simulink model "ScriptDemo"  (R2022b)
settings: configuration reference "TmVcThermal_Configuration_sub" (kept outside this file)
undefined symbols (not defined in the file): aaaa, bbbb, cTmComprCtrl_D_u8HvacFlowTable_db, cTmComprCtrl_D_u8HvacFlowTable_sw, cTmComprCtrl_n_i16ChillCmpIMax, cTmComprCtrl_n_i16ChillCmpIMin, cTmComprCtrl_n_i16ChillCmpIMin666, cTmComprCtrl_n_i16ChillCmpPMax, cTmComprCtrl_n_i16ChillCmpPMin, cTmComprCtrl_n_i16CmpChillCoolRpmKiMax, cTmComprCtrl_n_i16CmpChillCoolRpmKiMin, cTmComprCtrl_n_i16CmpChillCoolRpmKpMax, cTmComprCtrl_n_i16CmpChillCoolRpmKpMin, cTmComprCtrl_n_i16CmpCoolRpmKiMax, cTmComprCtrl_n_i16CmpCoolRpmKiMin, cTmComprCtrl_n_i16CmpCoolRpmKpMax, cTmComprCtrl_n_i16CmpCoolRpmKpMin, cTmComprCtrl_n_i16SM4CmpHeatKiMax, cTmComprCtrl_n_i16SM4CmpHeatKiMin, cTmComprCtrl_n_i16SM4CmpHeatKpMax, cTmComprCtrl_n_i16SM4CmpHeatKpMin, cTmComprCtrl_n_i16SM5CmpHeatKiMax, cTmComprCtrl_n_i16SM5CmpHeatKiMin, cTmComprCtrl_n_i16SM5CmpHeatKpMax, cTmComprCtrl_n_i16SM5CmpHeatKpMin, cTmComprCtrl_n_i16SM6CmpHeatKiMax, cTmComprCtrl_n_i16SM6CmpHeatKiMin, cTmComprCtrl_n_i16SM6CmpHeatKpMax, cTmComprCtrl_n_i16SM6CmpHeatKpMin, cTmComprCtrl_n_u16CmpMaxSpdFanFltLimt, cTmComprCtrl_n_u16CmpMaxSpdLoSidePFltLimt, cTmComprCtrl_n_u16CmpMaxSpdSensorFltLimt, cTmComprCtrl_n_u16CompMinRpm, cTmComprCtrl_n_u16CompRpmIncThres, cTmComprCtrl_t_u16BattCooltFFPeriod, cTmComprCtrl_t_u16BattCooltPIPeriod, cTmComprCtrl_t_u16CmpCoolFFPeriod, cTmComprCtrl_t_u16CmpCoolPIPeriod, cTmComprCtrl_t_u16CoolCmpChillFFPeriod, cTmComprCtrl_t_u16CoolCmpChillPIPeriod, cTmComprCtrl_t_u16SM4CmpHeatFFPeriod, cTmComprCtrl_t_u16SM4CmpHeatPIPeriod, cTmComprCtrl_t_u16SM5CmpHeatFFPeriod, cTmComprCtrl_t_u16SM5CmpHeatPIPeriod, cTmComprCtrl_t_u16SM6CmpHeatFFPeriod, cTmComprCtrl_t_u16SM6CmpHeatPIPeriod, cTmComprCtrl_Te_EvapClearInteg, cTmComprCtrl_Te_i16HpReqTempSaturoffset, cTmComprCtrl_Te_i16SatLpReplaceDiff, cTmComprCtrl_Te_i16SM3BatDiffStartEvapDecOffset, cTmComprCtrl_Te_i16SM3EvapLo, cTmComprCtrl_Te_i16SM3TBatDiffEntEvapDecOffset, cTmComprCtrl_Te_i16SM3TBatDiffEntEvapDecOffsetQuit, cTmComprCtrl_Te_s32ErrCmpChillPIContinueCoolH, cTmComprCtrl_Te_s32ErrCmpChillPIContinueCoolL, cTmComprCtrl_Te_s32ErrCmpPIContinueChillH, cTmComprCtrl_Te_s32ErrCmpPIContinueChillL, cTmComprCtrl_Te_s32ErrCmpPIContinueCoolH, cTmComprCtrl_Te_s32ErrCmpPIContinueCoolL, cTmComprCtrl_Te_s32ErrCmpPIContinueHeatH ... (+398)
libraries: simulink x782, PCMULib x640, simulink_need_slupdate x4
(part 9 of 41)

== system ScriptDemo/Create/Model/createModGotoAll/After ==
  note: createModGotoAll()
      |
      | # 在此路径下执行
  AFFaultLimit : Subsystem
  LoSidePFltLimt : Subsystem
  SensFaultLimit : Subsystem
  TAmbLimit : Subsystem
  wires:
  [sTmDiag_D_u8FanFltSt] -> AFFaultLimit/1(sTmDiag_D_u8FanFltSt)
  AFFaultLimit/1(rTmComprCtrl_n_u16CompMaxRpmAfFlt) -> [rTmComprCtrl_n_u16CompMaxRpmAfFlt]
  AFFaultLimit/2(xTmComprCtrl_B_CmpFanFltLimtFlag) -> [xTmComprCtrl_B_CmpFanFltLimtFlag]
  [sTmDiag_D_u8LoSidePFltSt] -> LoSidePFltLimt/1(sTmDiag_D_u8LoSidePFltSt)
  [sTmSigProces_Te_s32TAmb] -> LoSidePFltLimt/2(sTmSigProces_Te_s32TAmb)
  [sTmIn_D_u8HeatPump] -> LoSidePFltLimt/3(sTmIn_D_u8HeatPump)
  LoSidePFltLimt/1(rTmComprCtrl_n_u16CompMaxRpmLoSidePFlt) -> [rTmComprCtrl_n_u16CompMaxRpmLoSidePFlt]
  LoSidePFltLimt/2(xTmComprCtrl_B_CmpLoSidePFltLimtFlag) -> [xTmComprCtrl_B_CmpLoSidePFltLimtFlag]
  [sTmDiag_D_u8CmprDischrgTFltSt] -> SensFaultLimit/1(sTmDiag_D_u8CmprDischrgTFltSt)
  [sTmDiag_D_u8HiSidePFltSt] -> SensFaultLimit/2(sTmDiag_D_u8HiSidePFltSt)
  [sTmDiag_D_u8OutrCondOutTFltSt] -> SensFaultLimit/3(sTmDiag_D_u8OutrCondOutTFltSt)
  [sTmIn_D_u8HeatPump] -> SensFaultLimit/4(sTmIn_D_u8HeatPump)
  [sTmDiag_D_u8HiSidePNHPFltSt] -> SensFaultLimit/5(sTmDiag_D_u8HiSidePNHPFltSt)
  SensFaultLimit/1(rTmComprCtrl_n_u16CompMaxRpmSensFlt) -> [rTmComprCtrl_n_u16CompMaxRpmSensFlt]
  SensFaultLimit/2(xTmComprCtrl_B_CmpSensorFltLimtFlag) -> [xTmComprCtrl_B_CmpSensorFltLimtFlag]
  [sTmSigProces_Pw_i16ReqPwrForHeat] -> TAmbLimit/1(sTmSigProces_Pw_i16ReqPwrForHeat)
  [sTmSigProces_Te_s32TAmb] -> TAmbLimit/2(sTmSigProces_Te_s32TAmb)
  [rTmComprCtrl_n_u16CompRpmReqBoundary] -> TAmbLimit/3(rTmComprCtrl_n_u16CompRpmReqBoundary)
  [sTmRefriModeMgr_D_u8HPCurMode] -> TAmbLimit/4(sTmRefriModeMgr_D_u8HPCurMode)
  TAmbLimit/1(rTmComprCtrl_n_u16CompMaxRpmTAmb) -> [rTmComprCtrl_n_u16CompMaxRpmTAmb]
  TAmbLimit/2(xTmComprCtrl_B_CmpAmbLimtFlag) -> [xTmComprCtrl_B_CmpAmbLimtFlag]

== system ScriptDemo/Create/Model/createModGotoAll/Before ==
  AFFaultLimit : Subsystem
  LoSidePFltLimt : Subsystem
  SensFaultLimit : Subsystem
  TAmbLimit : Subsystem

== system ScriptDemo/Create/Model/createModGroundTerm/After ==
  note: % 目的: 为输出端口创建debug 及对应的输入模块
      | [cnt] = createDebug(gcs)
  sTmRefriVlvCtrl_X_s32CEXVPosReqIn : Inport  OutDataTypeStr=single
  sTmRefriVlvCtrl_X_s32EEXVPosReqIn : Inport  Port=2  OutDataTypeStr=single
  sTmRefriVlvCtrl_X_s32BEXVPosReqIn : Inport  Port=3  OutDataTypeStr=single
  yTmRefriVlvCtrl_B_HpcCexvMovEnableIn : Inport  Port=4  OutDataTypeStr=boolean
  sTmRefriVlvCtrl_Z_u8CEXVInitStateIn : Inport  Port=5  OutDataTypeStr=uint8
  yTmRefriVlvCtrl_B_CexvCalibReqIn : Inport  Port=6  OutDataTypeStr=boolean
  yTmRefriVlvCtrl_B_HpcEexvMovEnableIn : Inport  Port=7  OutDataTypeStr=boolean
  sTmRefriVlvCtrl_Z_u8EEXVInitStateIn : Inport  Port=8  OutDataTypeStr=uint8
  yTmRefriVlvCtrl_B_EexvCalibReqIn : Inport  Port=9  OutDataTypeStr=boolean
  yTmRefriVlvCtrl_B_HpcBexvMovEnableIn : Inport  Port=10  OutDataTypeStr=boolean
  sTmRefriVlvCtrl_Z_u8BEXVInitStateIn : Inport  Port=11  OutDataTypeStr=uint8
  yTmRefriVlvCtrl_B_BexvCalibReqIn : Inport  Port=12  OutDataTypeStr=boolean
  sTmRefriVlvCtrl_X_s32SM3BexvMaxPosIn : Inport  Port=13  OutDataTypeStr=single
  yTmRefriVlvCtrl_B_EvapBattTLimBexvEnaIn : Inport  Port=14  OutDataTypeStr=boolean
  sTmRefriVlvCtrl_D_u8EexvRefriSwitchStIn : Inport  Port=15  OutDataTypeStr=uint8
  sTmRefriVlvCtrl_D_u8CexvRefriSwitchStIn : Inport  Port=16  OutDataTypeStr=uint8
  sTmRefriVlvCtrl_D_u8BexvRefriSwitchStIn : Inport  Port=17  OutDataTypeStr=uint8
  OutDebug : PCMULib/Interface/OutdebugRvs  SWI=cTmRefriVlvCtrl_X_s32CEXVPosReq_sw  DBI=cTmRefriVlvCtrl_X_s32CEXVPosReq_db
      settings: SourceProductName=PCMULib
  OutDebug1 : PCMULib/Interface/OutdebugRvs  SWI=cTmRefriVlvCtrl_X_s32EEXVPosReq_sw  DBI=cTmRefriVlvCtrl_X_s32EEXVPosReq_db
      settings: SourceProductName=PCMULib
  OutDebug10 : PCMULib/Interface/OutdebugRvs  SWI=cTmRefriVlvCtrl_Z_u8BEXVInitState_sw  DBI=cTmRefriVlvCtrl_Z_u8BEXVInitState_db
      settings: SourceProductName=PCMULib
  OutDebug11 : PCMULib/Interface/OutdebugRvs  SWI=cTmRefriVlvCtrl_B_BexvCalibReq_sw  DBI=cTmRefriVlvCtrl_B_BexvCalibReq_db
      settings: SourceProductName=PCMULib
  OutDebug12 : PCMULib/Interface/OutdebugRvs  SWI=cTmRefriVlvCtrl_X_s32SM3BexvMaxPos_sw  DBI=cTmRefriVlvCtrl_X_s32SM3BexvMaxPos_db
      settings: SourceProductName=PCMULib
  OutDebug13 : PCMULib/Interface/OutdebugRvs  SWI=cTmRefriVlvCtrl_B_EvapBattTLimBexvEna_sw  DBI=cTmRefriVlvCtrl_B_EvapBattTLimBexvEna_db
      settings: SourceProductName=PCMULib
  OutDebug14 : PCMULib/Interface/OutdebugRvs  SWI=cTmRefriVlvCtrl_D_u8EexvRefriSwitchSt_sw  DBI=cTmRefriVlvCtrl_D_u8EexvRefriSwitchSt_db
      settings: SourceProductName=PCMULib
  OutDebug15 : PCMULib/Interface/OutdebugRvs  SWI=cTmRefriVlvCtrl_D_u8CexvRefriSwitchSt_sw  DBI=cTmRefriVlvCtrl_D_u8CexvRefriSwitchSt_db
      settings: SourceProductName=PCMULib
  OutDebug16 : PCMULib/Interface/OutdebugRvs  SWI=cTmRefriVlvCtrl_D_u8BexvRefriSwitchSt_sw  DBI=cTmRefriVlvCtrl_D_u8BexvRefriSwitchSt_db
      settings: SourceProductName=PCMULib
  OutDebug2 : PCMULib/Interface/OutdebugRvs  SWI=cTmRefriVlvCtrl_X_s32BEXVPosReq_sw  DBI=cTmRefriVlvCtrl_X_s32BEXVPosReq_db
      settings: SourceProductName=PCMULib
  OutDebug3 : PCMULib/Interface/OutdebugRvs  SWI=cTmRefriVlvCtrl_B_HpcCexvMovEnable_sw  DBI=cTmRefriVlvCtrl_B_HpcCexvMovEnable_db
      settings: SourceProductName=PCMULib
  OutDebug4 : PCMULib/Interface/OutdebugRvs  SWI=cTmRefriVlvCtrl_Z_u8CEXVInitState_sw  DBI=cTmRefriVlvCtrl_Z_u8CEXVInitState_db
      settings: SourceProductName=PCMULib
  OutDebug5 : PCMULib/Interface/OutdebugRvs  SWI=cTmRefriVlvCtrl_B_CexvCalibReq_sw  DBI=cTmRefriVlvCtrl_B_CexvCalibReq_db
      settings: SourceProductName=PCMULib
  OutDebug6 : PCMULib/Interface/OutdebugRvs  SWI=cTmRefriVlvCtrl_B_HpcEexvMovEnable_sw  DBI=cTmRefriVlvCtrl_B_HpcEexvMovEnable_db
      settings: SourceProductName=PCMULib
  OutDebug7 : PCMULib/Interface/OutdebugRvs  SWI=cTmRefriVlvCtrl_Z_u8EEXVInitState_sw  DBI=cTmRefriVlvCtrl_Z_u8EEXVInitState_db
      settings: SourceProductName=PCMULib
  OutDebug8 : PCMULib/Interface/OutdebugRvs  SWI=cTmRefriVlvCtrl_B_EexvCalibReq_sw  DBI=cTmRefriVlvCtrl_B_EexvCalibReq_db
      settings: SourceProductName=PCMULib
  OutDebug9 : PCMULib/Interface/OutdebugRvs  SWI=cTmRefriVlvCtrl_B_HpcBexvMovEnable_sw  DBI=cTmRefriVlvCtrl_B_HpcBexvMovEnable_db
      settings: SourceProductName=PCMULib
  sTmRefriVlvCtrl_X_s32CEXVPosReq : Outport  OutDataTypeStr=single
  sTmRefriVlvCtrl_X_s32EEXVPosReq : Outport  Port=2  OutDataTypeStr=single
  sTmRefriVlvCtrl_X_s32BEXVPosReq : Outport  Port=3  OutDataTypeStr=single
  yTmRefriVlvCtrl_B_HpcCexvMovEnable : Outport  Port=4  OutDataTypeStr=boolean
  sTmRefriVlvCtrl_Z_u8CEXVInitState : Outport  Port=5  OutDataTypeStr=uint8
  yTmRefriVlvCtrl_B_CexvCalibReq : Outport  Port=6  OutDataTypeStr=boolean
  yTmRefriVlvCtrl_B_HpcEexvMovEnable : Outport  Port=7  OutDataTypeStr=boolean
  sTmRefriVlvCtrl_Z_u8EEXVInitState : Outport  Port=8  OutDataTypeStr=uint8
  yTmRefriVlvCtrl_B_EexvCalibReq : Outport  Port=9  OutDataTypeStr=boolean
  yTmRefriVlvCtrl_B_HpcBexvMovEnable : Outport  Port=10  OutDataTypeStr=boolean
  sTmRefriVlvCtrl_Z_u8BEXVInitState : Outport  Port=11  OutDataTypeStr=uint8
  yTmRefriVlvCtrl_B_BexvCalibReq : Outport  Port=12  OutDataTypeStr=boolean
  sTmRefriVlvCtrl_X_s32SM3BexvMaxPos : Outport  Port=13  OutDataTypeStr=single
  yTmRefriVlvCtrl_B_EvapBattTLimBexvEna : Outport  Port=14  OutDataTypeStr=boolean
  sTmRefriVlvCtrl_D_u8EexvRefriSwitchSt : Outport  Port=15  OutDataTypeStr=uint8
  sTmRefriVlvCtrl_D_u8CexvRefriSwitchSt : Outport  Port=16  OutDataTypeStr=uint8
  sTmRefriVlvCtrl_D_u8BexvRefriSwitchSt : Outport  Port=17  OutDataTypeStr=uint8
  wires:
  sTmRefriVlvCtrl_X_s32SM3BexvMaxPosIn/1 -> OutDebug12/1
  OutDebug12/1 -> sTmRefriVlvCtrl_X_s32SM3BexvMaxPos/1
  sTmRefriVlvCtrl_X_s32BEXVPosReqIn/1 -> OutDebug2/1
  OutDebug2/1 -> sTmRefriVlvCtrl_X_s32BEXVPosReq/1
  OutDebug16/1 -> sTmRefriVlvCtrl_D_u8BexvRefriSwitchSt/1
  sTmRefriVlvCtrl_D_u8EexvRefriSwitchStIn/1 -> OutDebug14/1
  OutDebug5/1 -> yTmRefriVlvCtrl_B_CexvCalibReq/1
  OutDebug3/1 -> yTmRefriVlvCtrl_B_HpcCexvMovEnable/1
  sTmRefriVlvCtrl_Z_u8CEXVInitStateIn/1 -> OutDebug4/1
  OutDebug4/1 -> sTmRefriVlvCtrl_Z_u8CEXVInitState/1
  sTmRefriVlvCtrl_D_u8BexvRefriSwitchStIn/1 -> OutDebug16/1
  OutDebug1/1 -> sTmRefriVlvCtrl_X_s32EEXVPosReq/1
  OutDebug14/1 -> sTmRefriVlvCtrl_D_u8EexvRefriSwitchSt/1
  yTmRefriVlvCtrl_B_CexvCalibReqIn/1 -> OutDebug5/1
  sTmRefriVlvCtrl_X_s32EEXVPosReqIn/1 -> OutDebug1/1
  yTmRefriVlvCtrl_B_HpcCexvMovEnableIn/1 -> OutDebug3/1
  yTmRefriVlvCtrl_B_EvapBattTLimBexvEnaIn/1 -> OutDebug13/1
  OutDebug13/1 -> yTmRefriVlvCtrl_B_EvapBattTLimBexvEna/1
  sTmRefriVlvCtrl_Z_u8BEXVInitStateIn/1 -> OutDebug10/1
  OutDebug10/1 -> sTmRefriVlvCtrl_Z_u8BEXVInitState/1
  sTmRefriVlvCtrl_D_u8CexvRefriSwitchStIn/1 -> OutDebug15/1
  OutDebug15/1 -> sTmRefriVlvCtrl_D_u8CexvRefriSwitchSt/1
  OutDebug/1 -> sTmRefriVlvCtrl_X_s32CEXVPosReq/1
  OutDebug7/1 -> sTmRefriVlvCtrl_Z_u8EEXVInitState/1
  OutDebug8/1 -> yTmRefriVlvCtrl_B_EexvCalibReq/1
  yTmRefriVlvCtrl_B_EexvCalibReqIn/1 -> OutDebug8/1
  sTmRefriVlvCtrl_X_s32CEXVPosReqIn/1 -> OutDebug/1
  OutDebug6/1 -> yTmRefriVlvCtrl_B_HpcEexvMovEnable/1
  yTmRefriVlvCtrl_B_HpcEexvMovEnableIn/1 -> OutDebug6/1
  sTmRefriVlvCtrl_Z_u8EEXVInitStateIn/1 -> OutDebug7/1
  yTmRefriVlvCtrl_B_HpcBexvMovEnableIn/1 -> OutDebug9/1
  OutDebug9/1 -> yTmRefriVlvCtrl_B_HpcBexvMovEnable/1
  yTmRefriVlvCtrl_B_BexvCalibReqIn/1 -> OutDebug11/1
  OutDebug11/1 -> yTmRefriVlvCtrl_B_BexvCalibReq/1

== system ScriptDemo/Create/Model/createModGroundTerm/Before ==
  note: % 目的: 为输出端口创建debug 及对应的输入模块
      | [cnt] = createDebug(gcs)
  sTmRefriVlvCtrl_X_s32CEXVPosReqIn : Inport  OutDataTypeStr=single
  sTmRefriVlvCtrl_X_s32EEXVPosReqIn : Inport  Port=2  OutDataTypeStr=single
  sTmRefriVlvCtrl_X_s32BEXVPosReqIn : Inport  Port=3  OutDataTypeStr=single
  yTmRefriVlvCtrl_B_HpcCexvMovEnableIn : Inport  Port=4  OutDataTypeStr=boolean
  sTmRefriVlvCtrl_Z_u8CEXVInitStateIn : Inport  Port=5  OutDataTypeStr=uint8
  yTmRefriVlvCtrl_B_CexvCalibReqIn : Inport  Port=6  OutDataTypeStr=boolean
  yTmRefriVlvCtrl_B_HpcEexvMovEnableIn : Inport  Port=7  OutDataTypeStr=boolean
  sTmRefriVlvCtrl_Z_u8EEXVInitStateIn : Inport  Port=8  OutDataTypeStr=uint8
  yTmRefriVlvCtrl_B_EexvCalibReqIn : Inport  Port=9  OutDataTypeStr=boolean
  yTmRefriVlvCtrl_B_HpcBexvMovEnableIn : Inport  Port=10  OutDataTypeStr=boolean
  sTmRefriVlvCtrl_Z_u8BEXVInitStateIn : Inport  Port=11  OutDataTypeStr=uint8
  yTmRefriVlvCtrl_B_BexvCalibReqIn : Inport  Port=12  OutDataTypeStr=boolean
  sTmRefriVlvCtrl_X_s32SM3BexvMaxPosIn : Inport  Port=13  OutDataTypeStr=single
  yTmRefriVlvCtrl_B_EvapBattTLimBexvEnaIn : Inport  Port=14  OutDataTypeStr=boolean
  sTmRefriVlvCtrl_D_u8EexvRefriSwitchStIn : Inport  Port=15  OutDataTypeStr=uint8
  sTmRefriVlvCtrl_D_u8CexvRefriSwitchStIn : Inport  Port=16  OutDataTypeStr=uint8
  sTmRefriVlvCtrl_D_u8BexvRefriSwitchStIn : Inport  Port=17  OutDataTypeStr=uint8
  OutDebug : PCMULib/Interface/OutdebugRvs  SWI=cTmRefriVlvCtrl_X_s32CEXVPosReq_sw  DBI=cTmRefriVlvCtrl_X_s32CEXVPosReq_db
      settings: SourceProductName=PCMULib
  OutDebug1 : PCMULib/Interface/OutdebugRvs  SWI=cTmRefriVlvCtrl_X_s32EEXVPosReq_sw  DBI=cTmRefriVlvCtrl_X_s32EEXVPosReq_db
      settings: SourceProductName=PCMULib
  OutDebug10 : PCMULib/Interface/OutdebugRvs  SWI=cTmRefriVlvCtrl_Z_u8BEXVInitState_sw  DBI=cTmRefriVlvCtrl_Z_u8BEXVInitState_db
      settings: SourceProductName=PCMULib
  OutDebug11 : PCMULib/Interface/OutdebugRvs  SWI=cTmRefriVlvCtrl_B_BexvCalibReq_sw  DBI=cTmRefriVlvCtrl_B_BexvCalibReq_db
      settings: SourceProductName=PCMULib
  OutDebug12 : PCMULib/Interface/OutdebugRvs  SWI=cTmRefriVlvCtrl_X_s32SM3BexvMaxPos_sw  DBI=cTmRefriVlvCtrl_X_s32SM3BexvMaxPos_db
      settings: SourceProductName=PCMULib
  OutDebug13 : PCMULib/Interface/OutdebugRvs  SWI=cTmRefriVlvCtrl_B_EvapBattTLimBexvEna_sw  DBI=cTmRefriVlvCtrl_B_EvapBattTLimBexvEna_db
      settings: SourceProductName=PCMULib
  OutDebug14 : PCMULib/Interface/OutdebugRvs  SWI=cTmRefriVlvCtrl_D_u8EexvRefriSwitchSt_sw  DBI=cTmRefriVlvCtrl_D_u8EexvRefriSwitchSt_db
      settings: SourceProductName=PCMULib
  OutDebug15 : PCMULib/Interface/OutdebugRvs  SWI=cTmRefriVlvCtrl_D_u8CexvRefriSwitchSt_sw  DBI=cTmRefriVlvCtrl_D_u8CexvRefriSwitchSt_db
      settings: SourceProductName=PCMULib
  OutDebug16 : PCMULib/Interface/OutdebugRvs  SWI=cTmRefriVlvCtrl_D_u8BexvRefriSwitchSt_sw  DBI=cTmRefriVlvCtrl_D_u8BexvRefriSwitchSt_db
      settings: SourceProductName=PCMULib
  OutDebug2 : PCMULib/Interface/OutdebugRvs  SWI=cTmRefriVlvCtrl_X_s32BEXVPosReq_sw  DBI=cTmRefriVlvCtrl_X_s32BEXVPosReq_db
      settings: SourceProductName=PCMULib
  OutDebug3 : PCMULib/Interface/OutdebugRvs  SWI=cTmRefriVlvCtrl_B_HpcCexvMovEnable_sw  DBI=cTmRefriVlvCtrl_B_HpcCexvMovEnable_db
      settings: SourceProductName=PCMULib
  OutDebug4 : PCMULib/Interface/OutdebugRvs  SWI=cTmRefriVlvCtrl_Z_u8CEXVInitState_sw  DBI=cTmRefriVlvCtrl_Z_u8CEXVInitState_db
      settings: SourceProductName=PCMULib
  OutDebug5 : PCMULib/Interface/OutdebugRvs  SWI=cTmRefriVlvCtrl_B_CexvCalibReq_sw  DBI=cTmRefriVlvCtrl_B_CexvCalibReq_db
      settings: SourceProductName=PCMULib
  OutDebug6 : PCMULib/Interface/OutdebugRvs  SWI=cTmRefriVlvCtrl_B_HpcEexvMovEnable_sw  DBI=cTmRefriVlvCtrl_B_HpcEexvMovEnable_db
      settings: SourceProductName=PCMULib
  OutDebug7 : PCMULib/Interface/OutdebugRvs  SWI=cTmRefriVlvCtrl_Z_u8EEXVInitState_sw  DBI=cTmRefriVlvCtrl_Z_u8EEXVInitState_db
      settings: SourceProductName=PCMULib
  OutDebug8 : PCMULib/Interface/OutdebugRvs  SWI=cTmRefriVlvCtrl_B_EexvCalibReq_sw  DBI=cTmRefriVlvCtrl_B_EexvCalibReq_db
      settings: SourceProductName=PCMULib
  OutDebug9 : PCMULib/Interface/OutdebugRvs  SWI=cTmRefriVlvCtrl_B_HpcBexvMovEnable_sw  DBI=cTmRefriVlvCtrl_B_HpcBexvMovEnable_db
      settings: SourceProductName=PCMULib
  sTmRefriVlvCtrl_X_s32CEXVPosReq : Outport  OutDataTypeStr=single
  sTmRefriVlvCtrl_X_s32EEXVPosReq : Outport  Port=2  OutDataTypeStr=single
  sTmRefriVlvCtrl_X_s32BEXVPosReq : Outport  Port=3  OutDataTypeStr=single
  yTmRefriVlvCtrl_B_HpcCexvMovEnable : Outport  Port=4  OutDataTypeStr=boolean
  sTmRefriVlvCtrl_Z_u8CEXVInitState : Outport  Port=5  OutDataTypeStr=uint8
  yTmRefriVlvCtrl_B_CexvCalibReq : Outport  Port=6  OutDataTypeStr=boolean
  yTmRefriVlvCtrl_B_HpcEexvMovEnable : Outport  Port=7  OutDataTypeStr=boolean
  sTmRefriVlvCtrl_Z_u8EEXVInitState : Outport  Port=8  OutDataTypeStr=uint8
  yTmRefriVlvCtrl_B_EexvCalibReq : Outport  Port=9  OutDataTypeStr=boolean
  yTmRefriVlvCtrl_B_HpcBexvMovEnable : Outport  Port=10  OutDataTypeStr=boolean
  sTmRefriVlvCtrl_Z_u8BEXVInitState : Outport  Port=11  OutDataTypeStr=uint8
  yTmRefriVlvCtrl_B_BexvCalibReq : Outport  Port=12  OutDataTypeStr=boolean
  sTmRefriVlvCtrl_X_s32SM3BexvMaxPos : Outport  Port=13  OutDataTypeStr=single
  yTmRefriVlvCtrl_B_EvapBattTLimBexvEna : Outport  Port=14  OutDataTypeStr=boolean
  sTmRefriVlvCtrl_D_u8EexvRefriSwitchSt : Outport  Port=15  OutDataTypeStr=uint8
  sTmRefriVlvCtrl_D_u8CexvRefriSwitchSt : Outport  Port=16  OutDataTypeStr=uint8
  sTmRefriVlvCtrl_D_u8BexvRefriSwitchSt : Outport  Port=17  OutDataTypeStr=uint8
  wires:
  sTmRefriVlvCtrl_X_s32SM3BexvMaxPosIn/1 -> OutDebug12/1
  OutDebug12/1 -> sTmRefriVlvCtrl_X_s32SM3BexvMaxPos/1
  sTmRefriVlvCtrl_X_s32BEXVPosReqIn/1 -> OutDebug2/1
  OutDebug2/1 -> sTmRefriVlvCtrl_X_s32BEXVPosReq/1
  OutDebug16/1 -> sTmRefriVlvCtrl_D_u8BexvRefriSwitchSt/1
  sTmRefriVlvCtrl_D_u8EexvRefriSwitchStIn/1 -> OutDebug14/1
  OutDebug5/1 -> yTmRefriVlvCtrl_B_CexvCalibReq/1
  OutDebug3/1 -> yTmRefriVlvCtrl_B_HpcCexvMovEnable/1
  sTmRefriVlvCtrl_Z_u8CEXVInitStateIn/1 -> OutDebug4/1
  OutDebug4/1 -> sTmRefriVlvCtrl_Z_u8CEXVInitState/1
  sTmRefriVlvCtrl_D_u8BexvRefriSwitchStIn/1 -> OutDebug16/1
  OutDebug1/1 -> sTmRefriVlvCtrl_X_s32EEXVPosReq/1
  OutDebug14/1 -> sTmRefriVlvCtrl_D_u8EexvRefriSwitchSt/1
  yTmRefriVlvCtrl_B_CexvCalibReqIn/1 -> OutDebug5/1
  sTmRefriVlvCtrl_X_s32EEXVPosReqIn/1 -> OutDebug1/1
  yTmRefriVlvCtrl_B_HpcCexvMovEnableIn/1 -> OutDebug3/1
  yTmRefriVlvCtrl_B_EvapBattTLimBexvEnaIn/1 -> OutDebug13/1
  OutDebug13/1 -> yTmRefriVlvCtrl_B_EvapBattTLimBexvEna/1
  sTmRefriVlvCtrl_Z_u8BEXVInitStateIn/1 -> OutDebug10/1
  OutDebug10/1 -> sTmRefriVlvCtrl_Z_u8BEXVInitState/1
  sTmRefriVlvCtrl_D_u8CexvRefriSwitchStIn/1 -> OutDebug15/1
  OutDebug15/1 -> sTmRefriVlvCtrl_D_u8CexvRefriSwitchSt/1
  OutDebug/1 -> sTmRefriVlvCtrl_X_s32CEXVPosReq/1
  OutDebug7/1 -> sTmRefriVlvCtrl_Z_u8EEXVInitState/1
  OutDebug8/1 -> yTmRefriVlvCtrl_B_EexvCalibReq/1
  yTmRefriVlvCtrl_B_EexvCalibReqIn/1 -> OutDebug8/1
  sTmRefriVlvCtrl_X_s32CEXVPosReqIn/1 -> OutDebug/1
  OutDebug6/1 -> yTmRefriVlvCtrl_B_HpcEexvMovEnable/1
  yTmRefriVlvCtrl_B_HpcEexvMovEnableIn/1 -> OutDebug6/1
  sTmRefriVlvCtrl_Z_u8EEXVInitStateIn/1 -> OutDebug7/1
  yTmRefriVlvCtrl_B_HpcBexvMovEnableIn/1 -> OutDebug9/1
  OutDebug9/1 -> yTmRefriVlvCtrl_B_HpcBexvMovEnable/1
  yTmRefriVlvCtrl_B_BexvCalibReqIn/1 -> OutDebug11/1
  OutDebug11/1 -> yTmRefriVlvCtrl_B_BexvCalibReq/1

== system ScriptDemo/Create/Model/createModPorts/After ==
  note: % 选中模型执行如下代码
      | [createdInport, createdOutport] = createModPorts(gcb)
      | % 范例：[createdInport, createdOutport] = createModPorts(gcb,'mode','inport'),
      | % 范例：[createdInport, createdOutport] = createModPorts(gcb,'mode','outport'),
      | % 范例：[createdInport, createdOutport] = createModPorts(gcb,'mode','both'),
  sTmRefriVlvCtrl_X_s32CEXVPosReqIn : Inport  OutDataTypeStr=single  OutputFunctionCall=on
  sTmRefriVlvCtrl_X_s32EEXVPosReqIn : Inport  Port=2  OutDataTypeStr=single
  sTmRefriVlvCtrl_X_s32BEXVPosReqIn : Inport  Port=3  OutDataTypeStr=single
  yTmRefriVlvCtrl_B_HpcCexvMovEnableIn : Inport  Port=4  OutDataTypeStr=boolean
  sTmRefriVlvCtrl_Z_u8CEXVInitStateIn : Inport  Port=5  OutDataTypeStr=uint8
  yTmRefriVlvCtrl_B_CexvCalibReqIn : Inport  Port=6  OutDataTypeStr=boolean
  yTmRefriVlvCtrl_B_HpcEexvMovEnableIn : Inport  Port=7  OutDataTypeStr=boolean
  sTmRefriVlvCtrl_Z_u8EEXVInitStateIn : Inport  Port=8  OutDataTypeStr=uint8
  yTmRefriVlvCtrl_B_EexvCalibReqIn : Inport  Port=9  OutDataTypeStr=boolean
  yTmRefriVlvCtrl_B_HpcBexvMovEnableIn : Inport  Port=10  OutDataTypeStr=boolean
  sTmRefriVlvCtrl_Z_u8BEXVInitStateIn : Inport  Port=11  OutDataTypeStr=uint8
  yTmRefriVlvCtrl_B_BexvCalibReqIn : Inport  Port=12  OutDataTypeStr=boolean
  sTmRefriVlvCtrl_X_s32SM3BexvMaxPosIn : Inport  Port=13  OutDataTypeStr=single
  yTmRefriVlvCtrl_B_EvapBattTLimBexvEnaIn : Inport  Port=14  OutDataTypeStr=boolean
  sTmRefriVlvCtrl_D_u8EexvRefriSwitchStIn : Inport  Port=15  OutDataTypeStr=uint8
  sTmRefriVlvCtrl_D_u8CexvRefriSwitchStIn : Inport  Port=16  OutDataTypeStr=uint8
  sTmRefriVlvCtrl_D_u8BexvRefriSwitchStIn : Inport  Port=17  OutDataTypeStr=uint8
  Before : Subsystem
  sTmRefriVlvCtrl_X_s32CEXVPosReq : Outport  OutDataTypeStr=single
  sTmRefriVlvCtrl_X_s32EEXVPosReq : Outport  Port=2  OutDataTypeStr=single
  sTmRefriVlvCtrl_X_s32BEXVPosReq : Outport  Port=3  OutDataTypeStr=single
  yTmRefriVlvCtrl_B_HpcCexvMovEnable : Outport  Port=4  OutDataTypeStr=boolean
  sTmRefriVlvCtrl_Z_u8CEXVInitState : Outport  Port=5  OutDataTypeStr=uint8
  yTmRefriVlvCtrl_B_CexvCalibReq : Outport  Port=6  OutDataTypeStr=boolean
  yTmRefriVlvCtrl_B_HpcEexvMovEnable : Outport  Port=7  OutDataTypeStr=boolean
  sTmRefriVlvCtrl_Z_u8EEXVInitState : Outport  Port=8  OutDataTypeStr=uint8
  yTmRefriVlvCtrl_B_EexvCalibReq : Outport  Port=9  OutDataTypeStr=boolean
  yTmRefriVlvCtrl_B_HpcBexvMovEnable : Outport  Port=10  OutDataTypeStr=boolean
  sTmRefriVlvCtrl_Z_u8BEXVInitState : Outport  Port=11  OutDataTypeStr=uint8
  yTmRefriVlvCtrl_B_BexvCalibReq : Outport  Port=12  OutDataTypeStr=boolean
  sTmRefriVlvCtrl_X_s32SM3BexvMaxPos : Outport  Port=13  OutDataTypeStr=single
  yTmRefriVlvCtrl_B_EvapBattTLimBexvEna : Outport  Port=14  OutDataTypeStr=boolean
  sTmRefriVlvCtrl_D_u8EexvRefriSwitchSt : Outport  Port=15  OutDataTypeStr=uint8
  sTmRefriVlvCtrl_D_u8CexvRefriSwitchSt : Outport  Port=16  OutDataTypeStr=uint8
  sTmRefriVlvCtrl_D_u8BexvRefriSwitchSt : Outport  Port=17  OutDataTypeStr=uint8
  wires:
  sTmRefriVlvCtrl_X_s32CEXVPosReqIn/1 -> Before/1(sTmRefriVlvCtrl_X_s32CEXVPosReqIn)
  sTmRefriVlvCtrl_X_s32EEXVPosReqIn/1 -> Before/2(sTmRefriVlvCtrl_X_s32EEXVPosReqIn)
  sTmRefriVlvCtrl_X_s32BEXVPosReqIn/1 -> Before/3(sTmRefriVlvCtrl_X_s32BEXVPosReqIn)
  yTmRefriVlvCtrl_B_HpcCexvMovEnableIn/1 -> Before/4(yTmRefriVlvCtrl_B_HpcCexvMovEnableIn)
  sTmRefriVlvCtrl_Z_u8CEXVInitStateIn/1 -> Before/5(sTmRefriVlvCtrl_Z_u8CEXVInitStateIn)
  yTmRefriVlvCtrl_B_CexvCalibReqIn/1 -> Before/6(yTmRefriVlvCtrl_B_CexvCalibReqIn)
  yTmRefriVlvCtrl_B_HpcEexvMovEnableIn/1 -> Before/7(yTmRefriVlvCtrl_B_HpcEexvMovEnableIn)
  sTmRefriVlvCtrl_Z_u8EEXVInitStateIn/1 -> Before/8(sTmRefriVlvCtrl_Z_u8EEXVInitStateIn)
  yTmRefriVlvCtrl_B_EexvCalibReqIn/1 -> Before/9(yTmRefriVlvCtrl_B_EexvCalibReqIn)
  yTmRefriVlvCtrl_B_HpcBexvMovEnableIn/1 -> Before/10(yTmRefriVlvCtrl_B_HpcBexvMovEnableIn)
  sTmRefriVlvCtrl_Z_u8BEXVInitStateIn/1 -> Before/11(sTmRefriVlvCtrl_Z_u8BEXVInitStateIn)
  yTmRefriVlvCtrl_B_BexvCalibReqIn/1 -> Before/12(yTmRefriVlvCtrl_B_BexvCalibReqIn)
  sTmRefriVlvCtrl_X_s32SM3BexvMaxPosIn/1 -> Before/13(sTmRefriVlvCtrl_X_s32SM3BexvMaxPosIn)
  yTmRefriVlvCtrl_B_EvapBattTLimBexvEnaIn/1 -> Before/14(yTmRefriVlvCtrl_B_EvapBattTLimBexvEnaIn)
  sTmRefriVlvCtrl_D_u8EexvRefriSwitchStIn/1 -> Before/15(sTmRefriVlvCtrl_D_u8EexvRefriSwitchStIn)
  sTmRefriVlvCtrl_D_u8CexvRefriSwitchStIn/1 -> Before/16(sTmRefriVlvCtrl_D_u8CexvRefriSwitchStIn)
  sTmRefriVlvCtrl_D_u8BexvRefriSwitchStIn/1 -> Before/17(sTmRefriVlvCtrl_D_u8BexvRefriSwitchStIn)
  Before/1(sTmRefriVlvCtrl_X_s32CEXVPosReq) -> sTmRefriVlvCtrl_X_s32CEXVPosReq/1
  Before/2(sTmRefriVlvCtrl_X_s32EEXVPosReq) -> sTmRefriVlvCtrl_X_s32EEXVPosReq/1
  Before/3(sTmRefriVlvCtrl_X_s32BEXVPosReq) -> sTmRefriVlvCtrl_X_s32BEXVPosReq/1
  Before/4(yTmRefriVlvCtrl_B_HpcCexvMovEnable) -> yTmRefriVlvCtrl_B_HpcCexvMovEnable/1
  Before/5(sTmRefriVlvCtrl_Z_u8CEXVInitState) -> sTmRefriVlvCtrl_Z_u8CEXVInitState/1
  Before/6(yTmRefriVlvCtrl_B_CexvCalibReq) -> yTmRefriVlvCtrl_B_CexvCalibReq/1
  Before/7(yTmRefriVlvCtrl_B_HpcEexvMovEnable) -> yTmRefriVlvCtrl_B_HpcEexvMovEnable/1
  Before/8(sTmRefriVlvCtrl_Z_u8EEXVInitState) -> sTmRefriVlvCtrl_Z_u8EEXVInitState/1
  Before/9(yTmRefriVlvCtrl_B_EexvCalibReq) -> yTmRefriVlvCtrl_B_EexvCalibReq/1
  Before/10(yTmRefriVlvCtrl_B_HpcBexvMovEnable) -> yTmRefriVlvCtrl_B_HpcBexvMovEnable/1
  Before/11(sTmRefriVlvCtrl_Z_u8BEXVInitState) -> sTmRefriVlvCtrl_Z_u8BEXVInitState/1
  Before/12(yTmRefriVlvCtrl_B_BexvCalibReq) -> yTmRefriVlvCtrl_B_BexvCalibReq/1
  Before/13(sTmRefriVlvCtrl_X_s32SM3BexvMaxPos) -> sTmRefriVlvCtrl_X_s32SM3BexvMaxPos/1
  Before/14(yTmRefriVlvCtrl_B_EvapBattTLimBexvEna) -> yTmRefriVlvCtrl_B_EvapBattTLimBexvEna/1
  Before/15(sTmRefriVlvCtrl_D_u8EexvRefriSwitchSt) -> sTmRefriVlvCtrl_D_u8EexvRefriSwitchSt/1
  Before/16(sTmRefriVlvCtrl_D_u8CexvRefriSwitchSt) -> sTmRefriVlvCtrl_D_u8CexvRefriSwitchSt/1
  Before/17(sTmRefriVlvCtrl_D_u8BexvRefriSwitchSt) -> sTmRefriVlvCtrl_D_u8BexvRefriSwitchSt/1

== system ScriptDemo/Create/Model/createModPorts/Before ==
  note: % 目的: 为输出端口创建debug 及对应的输入模块
      | [cnt] = createDebug(gcs)
  sTmRefriVlvCtrl_X_s32CEXVPosReqIn : Inport  OutDataTypeStr=single
  sTmRefriVlvCtrl_X_s32EEXVPosReqIn : Inport  Port=2  OutDataTypeStr=single
  sTmRefriVlvCtrl_X_s32BEXVPosReqIn : Inport  Port=3  OutDataTypeStr=single
  yTmRefriVlvCtrl_B_HpcCexvMovEnableIn : Inport  Port=4  OutDataTypeStr=boolean
  sTmRefriVlvCtrl_Z_u8CEXVInitStateIn : Inport  Port=5  OutDataTypeStr=uint8
  yTmRefriVlvCtrl_B_CexvCalibReqIn : Inport  Port=6  OutDataTypeStr=boolean
  yTmRefriVlvCtrl_B_HpcEexvMovEnableIn : Inport  Port=7  OutDataTypeStr=boolean
  sTmRefriVlvCtrl_Z_u8EEXVInitStateIn : Inport  Port=8  OutDataTypeStr=uint8
  yTmRefriVlvCtrl_B_EexvCalibReqIn : Inport  Port=9  OutDataTypeStr=boolean
  yTmRefriVlvCtrl_B_HpcBexvMovEnableIn : Inport  Port=10  OutDataTypeStr=boolean
  sTmRefriVlvCtrl_Z_u8BEXVInitStateIn : Inport  Port=11  OutDataTypeStr=uint8
  yTmRefriVlvCtrl_B_BexvCalibReqIn : Inport  Port=12  OutDataTypeStr=boolean
  sTmRefriVlvCtrl_X_s32SM3BexvMaxPosIn : Inport  Port=13  OutDataTypeStr=single
  yTmRefriVlvCtrl_B_EvapBattTLimBexvEnaIn : Inport  Port=14  OutDataTypeStr=boolean
  sTmRefriVlvCtrl_D_u8EexvRefriSwitchStIn : Inport  Port=15  OutDataTypeStr=uint8
  sTmRefriVlvCtrl_D_u8CexvRefriSwitchStIn : Inport  Port=16  OutDataTypeStr=uint8
  sTmRefriVlvCtrl_D_u8BexvRefriSwitchStIn : Inport  Port=17  OutDataTypeStr=uint8
  OutDebug : PCMULib/Interface/OutdebugRvs  SWI=cTmRefriVlvCtrl_X_s32CEXVPosReq_sw  DBI=cTmRefriVlvCtrl_X_s32CEXVPosReq_db
      settings: SourceProductName=PCMULib
  OutDebug1 : PCMULib/Interface/OutdebugRvs  SWI=cTmRefriVlvCtrl_X_s32EEXVPosReq_sw  DBI=cTmRefriVlvCtrl_X_s32EEXVPosReq_db
      settings: SourceProductName=PCMULib
  OutDebug10 : PCMULib/Interface/OutdebugRvs  SWI=cTmRefriVlvCtrl_Z_u8BEXVInitState_sw  DBI=cTmRefriVlvCtrl_Z_u8BEXVInitState_db
      settings: SourceProductName=PCMULib
  OutDebug11 : PCMULib/Interface/OutdebugRvs  SWI=cTmRefriVlvCtrl_B_BexvCalibReq_sw  DBI=cTmRefriVlvCtrl_B_BexvCalibReq_db
      settings: SourceProductName=PCMULib
  OutDebug12 : PCMULib/Interface/OutdebugRvs  SWI=cTmRefriVlvCtrl_X_s32SM3BexvMaxPos_sw  DBI=cTmRefriVlvCtrl_X_s32SM3BexvMaxPos_db
      settings: SourceProductName=PCMULib
  OutDebug13 : PCMULib/Interface/OutdebugRvs  SWI=cTmRefriVlvCtrl_B_EvapBattTLimBexvEna_sw  DBI=cTmRefriVlvCtrl_B_EvapBattTLimBexvEna_db
      settings: SourceProductName=PCMULib
  OutDebug14 : PCMULib/Interface/OutdebugRvs  SWI=cTmRefriVlvCtrl_D_u8EexvRefriSwitchSt_sw  DBI=cTmRefriVlvCtrl_D_u8EexvRefriSwitchSt_db
      settings: SourceProductName=PCMULib
  OutDebug15 : PCMULib/Interface/OutdebugRvs  SWI=cTmRefriVlvCtrl_D_u8CexvRefriSwitchSt_sw  DBI=cTmRefriVlvCtrl_D_u8CexvRefriSwitchSt_db
      settings: SourceProductName=PCMULib
  OutDebug16 : PCMULib/Interface/OutdebugRvs  SWI=cTmRefriVlvCtrl_D_u8BexvRefriSwitchSt_sw  DBI=cTmRefriVlvCtrl_D_u8BexvRefriSwitchSt_db
      settings: SourceProductName=PCMULib
  OutDebug2 : PCMULib/Interface/OutdebugRvs  SWI=cTmRefriVlvCtrl_X_s32BEXVPosReq_sw  DBI=cTmRefriVlvCtrl_X_s32BEXVPosReq_db
      settings: SourceProductName=PCMULib
  OutDebug3 : PCMULib/Interface/OutdebugRvs  SWI=cTmRefriVlvCtrl_B_HpcCexvMovEnable_sw  DBI=cTmRefriVlvCtrl_B_HpcCexvMovEnable_db
      settings: SourceProductName=PCMULib
  OutDebug4 : PCMULib/Interface/OutdebugRvs  SWI=cTmRefriVlvCtrl_Z_u8CEXVInitState_sw  DBI=cTmRefriVlvCtrl_Z_u8CEXVInitState_db
      settings: SourceProductName=PCMULib
  OutDebug5 : PCMULib/Interface/OutdebugRvs  SWI=cTmRefriVlvCtrl_B_CexvCalibReq_sw  DBI=cTmRefriVlvCtrl_B_CexvCalibReq_db
      settings: SourceProductName=PCMULib
  OutDebug6 : PCMULib/Interface/OutdebugRvs  SWI=cTmRefriVlvCtrl_B_HpcEexvMovEnable_sw  DBI=cTmRefriVlvCtrl_B_HpcEexvMovEnable_db
      settings: SourceProductName=PCMULib
  OutDebug7 : PCMULib/Interface/OutdebugRvs  SWI=cTmRefriVlvCtrl_Z_u8EEXVInitState_sw  DBI=cTmRefriVlvCtrl_Z_u8EEXVInitState_db
      settings: SourceProductName=PCMULib
  OutDebug8 : PCMULib/Interface/OutdebugRvs  SWI=cTmRefriVlvCtrl_B_EexvCalibReq_sw  DBI=cTmRefriVlvCtrl_B_EexvCalibReq_db
      settings: SourceProductName=PCMULib
  OutDebug9 : PCMULib/Interface/OutdebugRvs  SWI=cTmRefriVlvCtrl_B_HpcBexvMovEnable_sw  DBI=cTmRefriVlvCtrl_B_HpcBexvMovEnable_db
      settings: SourceProductName=PCMULib
  sTmRefriVlvCtrl_X_s32CEXVPosReq : Outport  OutDataTypeStr=single
  sTmRefriVlvCtrl_X_s32EEXVPosReq : Outport  Port=2  OutDataTypeStr=single
  sTmRefriVlvCtrl_X_s32BEXVPosReq : Outport  Port=3  OutDataTypeStr=single
  yTmRefriVlvCtrl_B_HpcCexvMovEnable : Outport  Port=4  OutDataTypeStr=boolean
  sTmRefriVlvCtrl_Z_u8CEXVInitState : Outport  Port=5  OutDataTypeStr=uint8
  yTmRefriVlvCtrl_B_CexvCalibReq : Outport  Port=6  OutDataTypeStr=boolean
  yTmRefriVlvCtrl_B_HpcEexvMovEnable : Outport  Port=7  OutDataTypeStr=boolean
  sTmRefriVlvCtrl_Z_u8EEXVInitState : Outport  Port=8  OutDataTypeStr=uint8
  yTmRefriVlvCtrl_B_EexvCalibReq : Outport  Port=9  OutDataTypeStr=boolean
  yTmRefriVlvCtrl_B_HpcBexvMovEnable : Outport  Port=10  OutDataTypeStr=boolean
  sTmRefriVlvCtrl_Z_u8BEXVInitState : Outport  Port=11  OutDataTypeStr=uint8
  yTmRefriVlvCtrl_B_BexvCalibReq : Outport  Port=12  OutDataTypeStr=boolean
  sTmRefriVlvCtrl_X_s32SM3BexvMaxPos : Outport  Port=13  OutDataTypeStr=single
  yTmRefriVlvCtrl_B_EvapBattTLimBexvEna : Outport  Port=14  OutDataTypeStr=boolean
  sTmRefriVlvCtrl_D_u8EexvRefriSwitchSt : Outport  Port=15  OutDataTypeStr=uint8
  sTmRefriVlvCtrl_D_u8CexvRefriSwitchSt : Outport  Port=16  OutDataTypeStr=uint8
  sTmRefriVlvCtrl_D_u8BexvRefriSwitchSt : Outport  Port=17  OutDataTypeStr=uint8
  wires:
  sTmRefriVlvCtrl_X_s32SM3BexvMaxPosIn/1 -> OutDebug12/1
  OutDebug12/1 -> sTmRefriVlvCtrl_X_s32SM3BexvMaxPos/1
  sTmRefriVlvCtrl_X_s32BEXVPosReqIn/1 -> OutDebug2/1
  OutDebug2/1 -> sTmRefriVlvCtrl_X_s32BEXVPosReq/1
  OutDebug16/1 -> sTmRefriVlvCtrl_D_u8BexvRefriSwitchSt/1
  sTmRefriVlvCtrl_D_u8EexvRefriSwitchStIn/1 -> OutDebug14/1
  OutDebug5/1 -> yTmRefriVlvCtrl_B_CexvCalibReq/1
  OutDebug3/1 -> yTmRefriVlvCtrl_B_HpcCexvMovEnable/1
  sTmRefriVlvCtrl_Z_u8CEXVInitStateIn/1 -> OutDebug4/1
  OutDebug4/1 -> sTmRefriVlvCtrl_Z_u8CEXVInitState/1
  sTmRefriVlvCtrl_D_u8BexvRefriSwitchStIn/1 -> OutDebug16/1
  OutDebug1/1 -> sTmRefriVlvCtrl_X_s32EEXVPosReq/1
  OutDebug14/1 -> sTmRefriVlvCtrl_D_u8EexvRefriSwitchSt/1
  yTmRefriVlvCtrl_B_CexvCalibReqIn/1 -> OutDebug5/1
  sTmRefriVlvCtrl_X_s32EEXVPosReqIn/1 -> OutDebug1/1
  yTmRefriVlvCtrl_B_HpcCexvMovEnableIn/1 -> OutDebug3/1
  yTmRefriVlvCtrl_B_EvapBattTLimBexvEnaIn/1 -> OutDebug13/1
  OutDebug13/1 -> yTmRefriVlvCtrl_B_EvapBattTLimBexvEna/1
  sTmRefriVlvCtrl_Z_u8BEXVInitStateIn/1 -> OutDebug10/1
  OutDebug10/1 -> sTmRefriVlvCtrl_Z_u8BEXVInitState/1
  sTmRefriVlvCtrl_D_u8CexvRefriSwitchStIn/1 -> OutDebug15/1
  OutDebug15/1 -> sTmRefriVlvCtrl_D_u8CexvRefriSwitchSt/1
  OutDebug/1 -> sTmRefriVlvCtrl_X_s32CEXVPosReq/1
  OutDebug7/1 -> sTmRefriVlvCtrl_Z_u8EEXVInitState/1
  OutDebug8/1 -> yTmRefriVlvCtrl_B_EexvCalibReq/1
  yTmRefriVlvCtrl_B_EexvCalibReqIn/1 -> OutDebug8/1
  sTmRefriVlvCtrl_X_s32CEXVPosReqIn/1 -> OutDebug/1
  OutDebug6/1 -> yTmRefriVlvCtrl_B_HpcEexvMovEnable/1
  yTmRefriVlvCtrl_B_HpcEexvMovEnableIn/1 -> OutDebug6/1
  sTmRefriVlvCtrl_Z_u8EEXVInitStateIn/1 -> OutDebug7/1
  yTmRefriVlvCtrl_B_HpcBexvMovEnableIn/1 -> OutDebug9/1
  OutDebug9/1 -> yTmRefriVlvCtrl_B_HpcBexvMovEnable/1
  yTmRefriVlvCtrl_B_BexvCalibReqIn/1 -> OutDebug11/1
  OutDebug11/1 -> yTmRefriVlvCtrl_B_BexvCalibReq/1

== system ScriptDemo/Create/Model/createModSig/After1 ==
  note: % 鼠标选中模型执行如下代码
      | createModSig(gcb,'resoveValue',true)
  sTmRefriVlvCtrl_X_s32CEXVPosReqIn : Inport  OutDataTypeStr=single  OutputFunctionCall=on
  sTmRefriVlvCtrl_X_s32EEXVPosReqIn : Inport  Port=2  OutDataTypeStr=single
  sTmRefriVlvCtrl_X_s32BEXVPosReqIn : Inport  Port=3  OutDataTypeStr=single
  yTmRefriVlvCtrl_B_HpcCexvMovEnableIn : Inport  Port=4  OutDataTypeStr=boolean
  sTmRefriVlvCtrl_Z_u8CEXVInitStateIn : Inport  Port=5  OutDataTypeStr=uint8
  yTmRefriVlvCtrl_B_CexvCalibReqIn : Inport  Port=6  OutDataTypeStr=boolean
  yTmRefriVlvCtrl_B_HpcEexvMovEnableIn : Inport  Port=7  OutDataTypeStr=boolean
  sTmRefriVlvCtrl_Z_u8EEXVInitStateIn : Inport  Port=8  OutDataTypeStr=uint8
  yTmRefriVlvCtrl_B_EexvCalibReqIn : Inport  Port=9  OutDataTypeStr=boolean
  yTmRefriVlvCtrl_B_HpcBexvMovEnableIn : Inport  Port=10  OutDataTypeStr=boolean
  sTmRefriVlvCtrl_Z_u8BEXVInitStateIn : Inport  Port=11  OutDataTypeStr=uint8
  yTmRefriVlvCtrl_B_BexvCalibReqIn : Inport  Port=12  OutDataTypeStr=boolean
  sTmRefriVlvCtrl_X_s32SM3BexvMaxPosIn : Inport  Port=13  OutDataTypeStr=single
  yTmRefriVlvCtrl_B_EvapBattTLimBexvEnaIn : Inport  Port=14  OutDataTypeStr=boolean
  sTmRefriVlvCtrl_D_u8EexvRefriSwitchStIn : Inport  Port=15  OutDataTypeStr=uint8
  sTmRefriVlvCtrl_D_u8CexvRefriSwitchStIn : Inport  Port=16  OutDataTypeStr=uint8
  sTmRefriVlvCtrl_D_u8BexvRefriSwitchStIn : Inport  Port=17  OutDataTypeStr=uint8
  Before : Subsystem
  sTmRefriVlvCtrl_X_s32CEXVPosReq : Outport  OutDataTypeStr=single
  sTmRefriVlvCtrl_X_s32EEXVPosReq : Outport  Port=2  OutDataTypeStr=single
  sTmRefriVlvCtrl_X_s32BEXVPosReq : Outport  Port=3  OutDataTypeStr=single
  yTmRefriVlvCtrl_B_HpcCexvMovEnable : Outport  Port=4  OutDataTypeStr=boolean
  sTmRefriVlvCtrl_Z_u8CEXVInitState : Outport  Port=5  OutDataTypeStr=uint8
  yTmRefriVlvCtrl_B_CexvCalibReq : Outport  Port=6  OutDataTypeStr=boolean
  yTmRefriVlvCtrl_B_HpcEexvMovEnable : Outport  Port=7  OutDataTypeStr=boolean
  sTmRefriVlvCtrl_Z_u8EEXVInitState : Outport  Port=8  OutDataTypeStr=uint8
  yTmRefriVlvCtrl_B_EexvCalibReq : Outport  Port=9  OutDataTypeStr=boolean
  yTmRefriVlvCtrl_B_HpcBexvMovEnable : Outport  Port=10  OutDataTypeStr=boolean
  sTmRefriVlvCtrl_Z_u8BEXVInitState : Outport  Port=11  OutDataTypeStr=uint8
  yTmRefriVlvCtrl_B_BexvCalibReq : Outport  Port=12  OutDataTypeStr=boolean
  sTmRefriVlvCtrl_X_s32SM3BexvMaxPos : Outport  Port=13  OutDataTypeStr=single
  yTmRefriVlvCtrl_B_EvapBattTLimBexvEna : Outport  Port=14  OutDataTypeStr=boolean
  sTmRefriVlvCtrl_D_u8EexvRefriSwitchSt : Outport  Port=15  OutDataTypeStr=uint8
  sTmRefriVlvCtrl_D_u8CexvRefriSwitchSt : Outport  Port=16  OutDataTypeStr=uint8
  sTmRefriVlvCtrl_D_u8BexvRefriSwitchSt : Outport  Port=17  OutDataTypeStr=uint8
  wires:
  sTmRefriVlvCtrl_X_s32BEXVPosReqIn/1 -> Before/3(sTmRefriVlvCtrl_X_s32BEXVPosReqIn)  "sTmRefriVlvCtrl_X_s32BEXVPosReqIn"
  sTmRefriVlvCtrl_X_s32SM3BexvMaxPosIn/1 -> Before/13(sTmRefriVlvCtrl_X_s32SM3BexvMaxPosIn)  "sTmRefriVlvCtrl_X_s32SM3BexvMaxPosIn"
  sTmRefriVlvCtrl_Z_u8BEXVInitStateIn/1 -> Before/11(sTmRefriVlvCtrl_Z_u8BEXVInitStateIn)  "sTmRefriVlvCtrl_Z_u8BEXVInitStateIn"
  sTmRefriVlvCtrl_D_u8CexvRefriSwitchStIn/1 -> Before/16(sTmRefriVlvCtrl_D_u8CexvRefriSwitchStIn)  "sTmRefriVlvCtrl_D_u8CexvRefriSwitchStIn"
  yTmRefriVlvCtrl_B_EvapBattTLimBexvEnaIn/1 -> Before/14(yTmRefriVlvCtrl_B_EvapBattTLimBexvEnaIn)  "yTmRefriVlvCtrl_B_EvapBattTLimBexvEnaIn"
  yTmRefriVlvCtrl_B_HpcEexvMovEnableIn/1 -> Before/7(yTmRefriVlvCtrl_B_HpcEexvMovEnableIn)  "yTmRefriVlvCtrl_B_HpcEexvMovEnableIn"
  Before/3(sTmRefriVlvCtrl_X_s32BEXVPosReq) -> sTmRefriVlvCtrl_X_s32BEXVPosReq/1  "sTmRefriVlvCtrl_X_s32BEXVPosReq"
  yTmRefriVlvCtrl_B_EexvCalibReqIn/1 -> Before/9(yTmRefriVlvCtrl_B_EexvCalibReqIn)  "yTmRefriVlvCtrl_B_EexvCalibReqIn"
  Before/8(sTmRefriVlvCtrl_Z_u8EEXVInitState) -> sTmRefriVlvCtrl_Z_u8EEXVInitState/1  "sTmRefriVlvCtrl_Z_u8EEXVInitState"
  sTmRefriVlvCtrl_Z_u8EEXVInitStateIn/1 -> Before/8(sTmRefriVlvCtrl_Z_u8EEXVInitStateIn)  "sTmRefriVlvCtrl_Z_u8EEXVInitStateIn"
  yTmRefriVlvCtrl_B_HpcBexvMovEnableIn/1 -> Before/10(yTmRefriVlvCtrl_B_HpcBexvMovEnableIn)  "yTmRefriVlvCtrl_B_HpcBexvMovEnableIn"
  yTmRefriVlvCtrl_B_BexvCalibReqIn/1 -> Before/12(yTmRefriVlvCtrl_B_BexvCalibReqIn)  "yTmRefriVlvCtrl_B_BexvCalibReqIn"
  Before/5(sTmRefriVlvCtrl_Z_u8CEXVInitState) -> sTmRefriVlvCtrl_Z_u8CEXVInitState/1  "sTmRefriVlvCtrl_Z_u8CEXVInitState"
  Before/4(yTmRefriVlvCtrl_B_HpcCexvMovEnable) -> yTmRefriVlvCtrl_B_HpcCexvMovEnable/1  "yTmRefriVlvCtrl_B_HpcCexvMovEnable"
  Before/6(yTmRefriVlvCtrl_B_CexvCalibReq) -> yTmRefriVlvCtrl_B_CexvCalibReq/1  "yTmRefriVlvCtrl_B_CexvCalibReq"
  sTmRefriVlvCtrl_X_s32EEXVPosReqIn/1 -> Before/2(sTmRefriVlvCtrl_X_s32EEXVPosReqIn)  "sTmRefriVlvCtrl_X_s32EEXVPosReqIn"
  sTmRefriVlvCtrl_X_s32CEXVPosReqIn/1 -> Before/1(sTmRefriVlvCtrl_X_s32CEXVPosReqIn)  "sTmRefriVlvCtrl_X_s32CEXVPosReqIn"
  yTmRefriVlvCtrl_B_CexvCalibReqIn/1 -> Before/6(yTmRefriVlvCtrl_B_CexvCalibReqIn)  "yTmRefriVlvCtrl_B_CexvCalibReqIn"
  sTmRefriVlvCtrl_Z_u8CEXVInitStateIn/1 -> Before/5(sTmRefriVlvCtrl_Z_u8CEXVInitStateIn)  "sTmRefriVlvCtrl_Z_u8CEXVInitStateIn"
  yTmRefriVlvCtrl_B_HpcCexvMovEnableIn/1 -> Before/4(yTmRefriVlvCtrl_B_HpcCexvMovEnableIn)  "yTmRefriVlvCtrl_B_HpcCexvMovEnableIn"
  sTmRefriVlvCtrl_D_u8BexvRefriSwitchStIn/1 -> Before/17(sTmRefriVlvCtrl_D_u8BexvRefriSwitchStIn)  "sTmRefriVlvCtrl_D_u8BexvRefriSwitchStIn"
  Before/12(yTmRefriVlvCtrl_B_BexvCalibReq) -> yTmRefriVlvCtrl_B_BexvCalibReq/1  "yTmRefriVlvCtrl_B_BexvCalibReq"
  Before/11(sTmRefriVlvCtrl_Z_u8BEXVInitState) -> sTmRefriVlvCtrl_Z_u8BEXVInitState/1  "sTmRefriVlvCtrl_Z_u8BEXVInitState"
  Before/1(sTmRefriVlvCtrl_X_s32CEXVPosReq) -> sTmRefriVlvCtrl_X_s32CEXVPosReq/1  "sTmRefriVlvCtrl_X_s32CEXVPosReq"
  Before/7(yTmRefriVlvCtrl_B_HpcEexvMovEnable) -> yTmRefriVlvCtrl_B_HpcEexvMovEnable/1  "yTmRefriVlvCtrl_B_HpcEexvMovEnable"
  sTmRefriVlvCtrl_D_u8EexvRefriSwitchStIn/1 -> Before/15(sTmRefriVlvCtrl_D_u8EexvRefriSwitchStIn)  "sTmRefriVlvCtrl_D_u8EexvRefriSwitchStIn"
  Before/10(yTmRefriVlvCtrl_B_HpcBexvMovEnable) -> yTmRefriVlvCtrl_B_HpcBexvMovEnable/1  "yTmRefriVlvCtrl_B_HpcBexvMovEnable"
  Before/14(yTmRefriVlvCtrl_B_EvapBattTLimBexvEna) -> yTmRefriVlvCtrl_B_EvapBattTLimBexvEna/1  "yTmRefriVlvCtrl_B_EvapBattTLimBexvEna"
  Before/9(yTmRefriVlvCtrl_B_EexvCalibReq) -> yTmRefriVlvCtrl_B_EexvCalibReq/1  "yTmRefriVlvCtrl_B_EexvCalibReq"
  Before/15(sTmRefriVlvCtrl_D_u8EexvRefriSwitchSt) -> sTmRefriVlvCtrl_D_u8EexvRefriSwitchSt/1  "sTmRefriVlvCtrl_D_u8EexvRefriSwitchSt"
  Before/13(sTmRefriVlvCtrl_X_s32SM3BexvMaxPos) -> sTmRefriVlvCtrl_X_s32SM3BexvMaxPos/1  "sTmRefriVlvCtrl_X_s32SM3BexvMaxPos"
  Before/17(sTmRefriVlvCtrl_D_u8BexvRefriSwitchSt) -> sTmRefriVlvCtrl_D_u8BexvRefriSwitchSt/1  "sTmRefriVlvCtrl_D_u8BexvRefriSwitchSt"
  Before/2(sTmRefriVlvCtrl_X_s32EEXVPosReq) -> sTmRefriVlvCtrl_X_s32EEXVPosReq/1  "sTmRefriVlvCtrl_X_s32EEXVPosReq"
  Before/16(sTmRefriVlvCtrl_D_u8CexvRefriSwitchSt) -> sTmRefriVlvCtrl_D_u8CexvRefriSwitchSt/1  "sTmRefriVlvCtrl_D_u8CexvRefriSwitchSt"

== system ScriptDemo/Create/Model/createModSig/After2 ==
  note: % 鼠标选中模型执行如下代码
      | createModSig(gcb,'logValue',true)
  sTmRefriVlvCtrl_X_s32CEXVPosReqIn : Inport  OutDataTypeStr=single  OutputFunctionCall=on
  sTmRefriVlvCtrl_X_s32EEXVPosReqIn : Inport  Port=2  OutDataTypeStr=single
  sTmRefriVlvCtrl_X_s32BEXVPosReqIn : Inport  Port=3  OutDataTypeStr=single
  yTmRefriVlvCtrl_B_HpcCexvMovEnableIn : Inport  Port=4  OutDataTypeStr=boolean
  sTmRefriVlvCtrl_Z_u8CEXVInitStateIn : Inport  Port=5  OutDataTypeStr=uint8
  yTmRefriVlvCtrl_B_CexvCalibReqIn : Inport  Port=6  OutDataTypeStr=boolean
  yTmRefriVlvCtrl_B_HpcEexvMovEnableIn : Inport  Port=7  OutDataTypeStr=boolean
  sTmRefriVlvCtrl_Z_u8EEXVInitStateIn : Inport  Port=8  OutDataTypeStr=uint8
  yTmRefriVlvCtrl_B_EexvCalibReqIn : Inport  Port=9  OutDataTypeStr=boolean
  yTmRefriVlvCtrl_B_HpcBexvMovEnableIn : Inport  Port=10  OutDataTypeStr=boolean
  sTmRefriVlvCtrl_Z_u8BEXVInitStateIn : Inport  Port=11  OutDataTypeStr=uint8
  yTmRefriVlvCtrl_B_BexvCalibReqIn : Inport  Port=12  OutDataTypeStr=boolean
  sTmRefriVlvCtrl_X_s32SM3BexvMaxPosIn : Inport  Port=13  OutDataTypeStr=single
  yTmRefriVlvCtrl_B_EvapBattTLimBexvEnaIn : Inport  Port=14  OutDataTypeStr=boolean
  sTmRefriVlvCtrl_D_u8EexvRefriSwitchStIn : Inport  Port=15  OutDataTypeStr=uint8
  sTmRefriVlvCtrl_D_u8CexvRefriSwitchStIn : Inport  Port=16  OutDataTypeStr=uint8
  sTmRefriVlvCtrl_D_u8BexvRefriSwitchStIn : Inport  Port=17  OutDataTypeStr=uint8
  Before : Subsystem
  sTmRefriVlvCtrl_X_s32CEXVPosReq : Outport  OutDataTypeStr=single
  sTmRefriVlvCtrl_X_s32EEXVPosReq : Outport  Port=2  OutDataTypeStr=single
  sTmRefriVlvCtrl_X_s32BEXVPosReq : Outport  Port=3  OutDataTypeStr=single
  yTmRefriVlvCtrl_B_HpcCexvMovEnable : Outport  Port=4  OutDataTypeStr=boolean
  sTmRefriVlvCtrl_Z_u8CEXVInitState : Outport  Port=5  OutDataTypeStr=uint8
  yTmRefriVlvCtrl_B_CexvCalibReq : Outport  Port=6  OutDataTypeStr=boolean
  yTmRefriVlvCtrl_B_HpcEexvMovEnable : Outport  Port=7  OutDataTypeStr=boolean
  sTmRefriVlvCtrl_Z_u8EEXVInitState : Outport  Port=8  OutDataTypeStr=uint8
  yTmRefriVlvCtrl_B_EexvCalibReq : Outport  Port=9  OutDataTypeStr=boolean
  yTmRefriVlvCtrl_B_HpcBexvMovEnable : Outport  Port=10  OutDataTypeStr=boolean
  sTmRefriVlvCtrl_Z_u8BEXVInitState : Outport  Port=11  OutDataTypeStr=uint8
  yTmRefriVlvCtrl_B_BexvCalibReq : Outport  Port=12  OutDataTypeStr=boolean
  sTmRefriVlvCtrl_X_s32SM3BexvMaxPos : Outport  Port=13  OutDataTypeStr=single
  yTmRefriVlvCtrl_B_EvapBattTLimBexvEna : Outport  Port=14  OutDataTypeStr=boolean
  sTmRefriVlvCtrl_D_u8EexvRefriSwitchSt : Outport  Port=15  OutDataTypeStr=uint8
  sTmRefriVlvCtrl_D_u8CexvRefriSwitchSt : Outport  Port=16  OutDataTypeStr=uint8
  sTmRefriVlvCtrl_D_u8BexvRefriSwitchSt : Outport  Port=17  OutDataTypeStr=uint8
  wires:
  sTmRefriVlvCtrl_X_s32BEXVPosReqIn/1 -> Before/3(sTmRefriVlvCtrl_X_s32BEXVPosReqIn)  "sTmRefriVlvCtrl_X_s32BEXVPosReqIn"
  sTmRefriVlvCtrl_X_s32SM3BexvMaxPosIn/1 -> Before/13(sTmRefriVlvCtrl_X_s32SM3BexvMaxPosIn)  "sTmRefriVlvCtrl_X_s32SM3BexvMaxPosIn"
  sTmRefriVlvCtrl_Z_u8BEXVInitStateIn/1 -> Before/11(sTmRefriVlvCtrl_Z_u8BEXVInitStateIn)  "sTmRefriVlvCtrl_Z_u8BEXVInitStateIn"
  sTmRefriVlvCtrl_D_u8CexvRefriSwitchStIn/1 -> Before/16(sTmRefriVlvCtrl_D_u8CexvRefriSwitchStIn)  "sTmRefriVlvCtrl_D_u8CexvRefriSwitchStIn"
  yTmRefriVlvCtrl_B_EvapBattTLimBexvEnaIn/1 -> Before/14(yTmRefriVlvCtrl_B_EvapBattTLimBexvEnaIn)  "yTmRefriVlvCtrl_B_EvapBattTLimBexvEnaIn"
  yTmRefriVlvCtrl_B_HpcEexvMovEnableIn/1 -> Before/7(yTmRefriVlvCtrl_B_HpcEexvMovEnableIn)  "yTmRefriVlvCtrl_B_HpcEexvMovEnableIn"
  Before/3(sTmRefriVlvCtrl_X_s32BEXVPosReq) -> sTmRefriVlvCtrl_X_s32BEXVPosReq/1  "sTmRefriVlvCtrl_X_s32BEXVPosReq"
  yTmRefriVlvCtrl_B_EexvCalibReqIn/1 -> Before/9(yTmRefriVlvCtrl_B_EexvCalibReqIn)  "yTmRefriVlvCtrl_B_EexvCalibReqIn"
  Before/8(sTmRefriVlvCtrl_Z_u8EEXVInitState) -> sTmRefriVlvCtrl_Z_u8EEXVInitState/1  "sTmRefriVlvCtrl_Z_u8EEXVInitState"
  sTmRefriVlvCtrl_Z_u8EEXVInitStateIn/1 -> Before/8(sTmRefriVlvCtrl_Z_u8EEXVInitStateIn)  "sTmRefriVlvCtrl_Z_u8EEXVInitStateIn"
  yTmRefriVlvCtrl_B_HpcBexvMovEnableIn/1 -> Before/10(yTmRefriVlvCtrl_B_HpcBexvMovEnableIn)  "yTmRefriVlvCtrl_B_HpcBexvMovEnableIn"
  yTmRefriVlvCtrl_B_BexvCalibReqIn/1 -> Before/12(yTmRefriVlvCtrl_B_BexvCalibReqIn)  "yTmRefriVlvCtrl_B_BexvCalibReqIn"
  Before/5(sTmRefriVlvCtrl_Z_u8CEXVInitState) -> sTmRefriVlvCtrl_Z_u8CEXVInitState/1  "sTmRefriVlvCtrl_Z_u8CEXVInitState"
  Before/4(yTmRefriVlvCtrl_B_HpcCexvMovEnable) -> yTmRefriVlvCtrl_B_HpcCexvMovEnable/1  "yTmRefriVlvCtrl_B_HpcCexvMovEnable"
  Before/6(yTmRefriVlvCtrl_B_CexvCalibReq) -> yTmRefriVlvCtrl_B_CexvCalibReq/1  "yTmRefriVlvCtrl_B_CexvCalibReq"
  sTmRefriVlvCtrl_X_s32EEXVPosReqIn/1 -> Before/2(sTmRefriVlvCtrl_X_s32EEXVPosReqIn)  "sTmRefriVlvCtrl_X_s32EEXVPosReqIn"
  sTmRefriVlvCtrl_X_s32CEXVPosReqIn/1 -> Before/1(sTmRefriVlvCtrl_X_s32CEXVPosReqIn)  "sTmRefriVlvCtrl_X_s32CEXVPosReqIn"
  yTmRefriVlvCtrl_B_CexvCalibReqIn/1 -> Before/6(yTmRefriVlvCtrl_B_CexvCalibReqIn)  "yTmRefriVlvCtrl_B_CexvCalibReqIn"
  sTmRefriVlvCtrl_Z_u8CEXVInitStateIn/1 -> Before/5(sTmRefriVlvCtrl_Z_u8CEXVInitStateIn)  "sTmRefriVlvCtrl_Z_u8CEXVInitStateIn"
  yTmRefriVlvCtrl_B_HpcCexvMovEnableIn/1 -> Before/4(yTmRefriVlvCtrl_B_HpcCexvMovEnableIn)  "yTmRefriVlvCtrl_B_HpcCexvMovEnableIn"
  sTmRefriVlvCtrl_D_u8BexvRefriSwitchStIn/1 -> Before/17(sTmRefriVlvCtrl_D_u8BexvRefriSwitchStIn)  "sTmRefriVlvCtrl_D_u8BexvRefriSwitchStIn"
  Before/12(yTmRefriVlvCtrl_B_BexvCalibReq) -> yTmRefriVlvCtrl_B_BexvCalibReq/1  "yTmRefriVlvCtrl_B_BexvCalibReq"
  Before/11(sTmRefriVlvCtrl_Z_u8BEXVInitState) -> sTmRefriVlvCtrl_Z_u8BEXVInitState/1  "sTmRefriVlvCtrl_Z_u8BEXVInitState"
  Before/1(sTmRefriVlvCtrl_X_s32CEXVPosReq) -> sTmRefriVlvCtrl_X_s32CEXVPosReq/1  "sTmRefriVlvCtrl_X_s32CEXVPosReq"
  Before/7(yTmRefriVlvCtrl_B_HpcEexvMovEnable) -> yTmRefriVlvCtrl_B_HpcEexvMovEnable/1  "yTmRefriVlvCtrl_B_HpcEexvMovEnable"
  sTmRefriVlvCtrl_D_u8EexvRefriSwitchStIn/1 -> Before/15(sTmRefriVlvCtrl_D_u8EexvRefriSwitchStIn)  "sTmRefriVlvCtrl_D_u8EexvRefriSwitchStIn"
  Before/10(yTmRefriVlvCtrl_B_HpcBexvMovEnable) -> yTmRefriVlvCtrl_B_HpcBexvMovEnable/1  "yTmRefriVlvCtrl_B_HpcBexvMovEnable"
  Before/14(yTmRefriVlvCtrl_B_EvapBattTLimBexvEna) -> yTmRefriVlvCtrl_B_EvapBattTLimBexvEna/1  "yTmRefriVlvCtrl_B_EvapBattTLimBexvEna"
  Before/9(yTmRefriVlvCtrl_B_EexvCalibReq) -> yTmRefriVlvCtrl_B_EexvCalibReq/1  "yTmRefriVlvCtrl_B_EexvCalibReq"
  Before/15(sTmRefriVlvCtrl_D_u8EexvRefriSwitchSt) -> sTmRefriVlvCtrl_D_u8EexvRefriSwitchSt/1  "sTmRefriVlvCtrl_D_u8EexvRefriSwitchSt"
  Before/13(sTmRefriVlvCtrl_X_s32SM3BexvMaxPos) -> sTmRefriVlvCtrl_X_s32SM3BexvMaxPos/1  "sTmRefriVlvCtrl_X_s32SM3BexvMaxPos"
  Before/17(sTmRefriVlvCtrl_D_u8BexvRefriSwitchSt) -> sTmRefriVlvCtrl_D_u8BexvRefriSwitchSt/1  "sTmRefriVlvCtrl_D_u8BexvRefriSwitchSt"
  Before/2(sTmRefriVlvCtrl_X_s32EEXVPosReq) -> sTmRefriVlvCtrl_X_s32EEXVPosReq/1  "sTmRefriVlvCtrl_X_s32EEXVPosReq"
  Before/16(sTmRefriVlvCtrl_D_u8CexvRefriSwitchSt) -> sTmRefriVlvCtrl_D_u8CexvRefriSwitchSt/1  "sTmRefriVlvCtrl_D_u8CexvRefriSwitchSt"
